simulink model "district_screening_model"  (R2026a)
settings: Solver=VariableStepAuto
values from neighbouring files (symbols this model uses):
  casesPerHourPerReviewer = 15    [build_simulink_workflow.m]
  gpuThroughputFactor = 0.98    [build_simulink_workflow.m]
  maxBandwidthImagesPerHour = 300    [build_simulink_workflow.m]
  numCameras = 4    [build_simulink_workflow.m]
  numOphthalmologists = 2    [build_simulink_workflow.m]

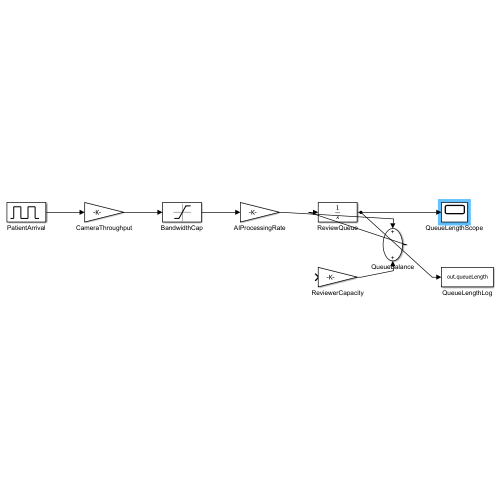
[thumbnail: Simulink's stored preview of the top-level diagram]
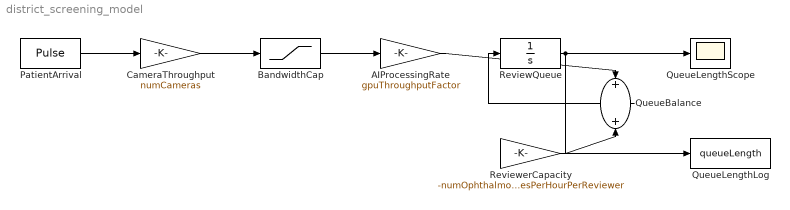
== system district_screening_model ==
  AIProcessingRate : Gain  Gain=gpuThroughputFactor
  BandwidthCap : Saturate  UpperLimit=maxBandwidthImagesPerHour  LowerLimit=0
  CameraThroughput : Gain  Gain=numCameras
  PatientArrival : DiscretePulseGenerator  PulseType=Time based  Period=1  PulseWidth=10
  QueueBalance : Sum
  QueueLengthLog : ToWorkspace  VariableName=queueLength  SaveFormat=Timeseries  SampleTime=-1
  QueueLengthScope : Scope
      settings: ActiveDisplayYMinimum=-0.62499999999999878  ActiveDisplayYMaximum=5.62499999999999
  ReviewQueue : Integrator
  ReviewerCapacity : Gain  Gain=-numOphthalmologists*casesPerHourPerReviewer
  wires:
  PatientArrival/1 -> CameraThroughput/1
  CameraThroughput/1 -> BandwidthCap/1
  BandwidthCap/1 -> AIProcessingRate/1
  AIProcessingRate/1 -> QueueBalance/1
  ReviewerCapacity/1 -> QueueBalance/2
  QueueBalance/1 -> ReviewQueue/1
  ReviewQueue/1 -> QueueLengthScope/1, QueueLengthLog/1
